simulink model "speed_control_rotativo_closed_loop"  (R2022b)
settings: Solver=VariableStepAuto  StartTime=0.0  StopTime=50  FixedStep=0.01  MaxStep=0.0005  RelTol=1e-3
libraries: simulink x5, autolibim x1, slpidlib x1
settings Model: Creator=mique  LastModifiedBy=mique

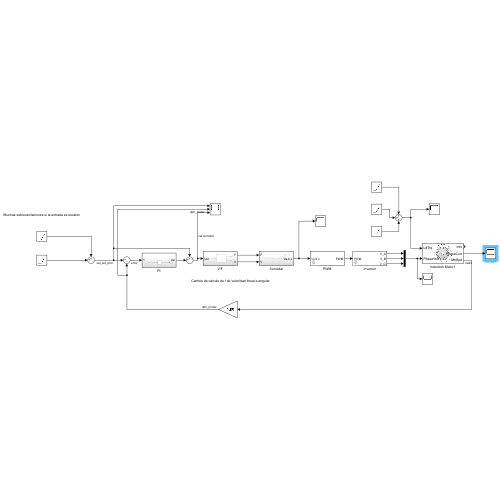
[thumbnail: Simulink's stored preview of the top-level diagram]
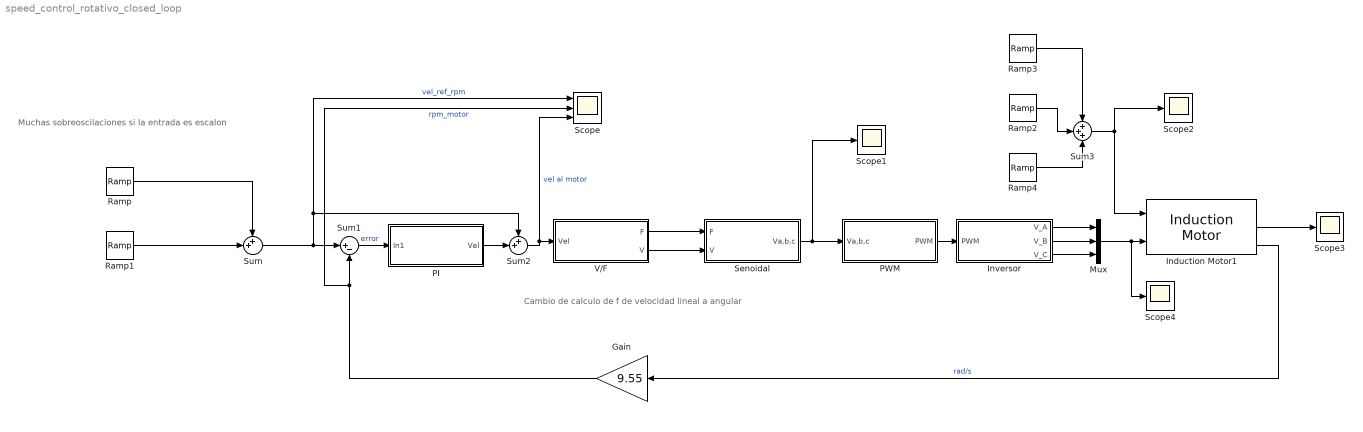
== system speed_control_rotativo_closed_loop ==
  note: Muchas sobreoscilaciones si la entrada es escalon
  note: Cambio de calculo de f de velocidad lineal a angular
  Gain : Gain  Gain=9.55
  Induction Motor1 : autolibim/Induction Motor  sim_type=Continuous  Ts=0.001  port_config=Torque  P=2  Zs=[1.77 0.0139]  Zr="[1.34  0.0121]"  Lm=0.3687  mechanical=[0.001 0 0]  theta_init=0  omega_init=0  RefBlkName='autolibim/Induction Motor'  aMode=5
      settings: LibrarySourceBlock=mcblib/Electrical Systems/Motors/Induction Motor
  Inversor : Subsystem  mask{Vmax=220}
      mask prompts: Vmax "Voltaje Maximo"
  Mux : Mux  Inputs=3
  PI : Subsystem
  PWM : Subsystem  mask{Vmax=220}
      mask prompts: Vmax "Voltaje Maximo"
  Ramp : simulink/Sources/Ramp  slope=-10  start=6  InitialOutput=0
  Ramp1 : simulink/Sources/Ramp  slope=10  start=0  InitialOutput=0
  Ramp2 : simulink/Sources/Ramp  slope=2  start=0.1  InitialOutput=0
  Ramp3 : simulink/Sources/Ramp  slope=-2  start=15  InitialOutput=0
  Ramp4 : simulink/Sources/Ramp  slope=-2  start=35  InitialOutput=0
  Scope : Scope  NumInputPorts=3
  Scope{1..4} (4 alike) : Scope
  Senoidal : Subsystem
  Sum : Sum  Inputs=++|
  Sum1 : Sum  Inputs=|+-
  Sum2 : Sum  Inputs=++|
  Sum3 : Sum  Inputs=+++
  V/F : Subsystem
  wires:
  V/F/1(F) -> Senoidal/1(F)
  Induction Motor1/2 -> Scope3/1
  Mux/1 -> Induction Motor1/2, Scope4/1
  Inversor/3(V_C) -> Mux/3
  Senoidal/1(Va,b,c) -> Scope1/1, PWM/1(Va,b,c)
  PWM/1(PWM) -> Inversor/1(PWM)
  Inversor/1(V_A) -> Mux/1
  Inversor/2(V_B) -> Mux/2
  V/F/2(V) -> Senoidal/2(V)
  Induction Motor1/3 -> Gain/1  "rad/s"
  Gain/1 -> Scope/2, Sum1/2  "rpm_motor"
  Sum/1 -> Sum2/1, Scope/1, Sum1/1  "vel_ref_rpm"
  Sum1/1 -> PI/1(In1)  "error"
  Sum2/1 -> V/F/1(Vel), Scope/3  "vel al motor"
  PI/1(Vel) -> Sum2/2
  Ramp1/1 -> Sum/2
  Ramp/1 -> Sum/1
  Ramp4/1 -> Sum3/3
  Ramp3/1 -> Sum3/1
  Sum3/1 -> Scope2/1, Induction Motor1/1
  Ramp2/1 -> Sum3/2

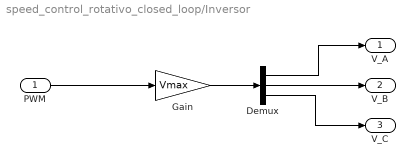
== system speed_control_rotativo_closed_loop/Inversor ==
  PWM : Inport
  Demux : Demux  Outputs=3
  Gain : Gain  Gain=Vmax
  V_A : Outport
  V_B : Outport  Port=2
  V_C : Outport  Port=3
  wires:
  PWM/1 -> Gain/1
  Demux/1 -> V_A/1
  Gain/1 -> Demux/1
  Demux/2 -> V_B/1
  Demux/3 -> V_C/1

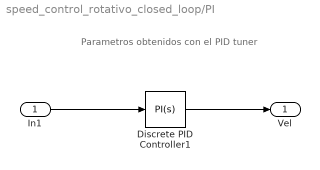
== system speed_control_rotativo_closed_loop/PI ==
  note: Parametros obtenidos con el PID tuner
  In1 : Inport
  Discrete PID Controller1 : slpidlib/PID Controller  Controller=PI  Form=Parallel  TimeDomain=Continuous-time  UseExternalTs=off  SampleTime=-1  IntegratorMethod=Forward Euler  FilterMethod=Forward Euler  ControllerParametersSource=internal  P=1  I=4.18069201960826  UseKiTs=off  D=0.0001  N=10  UseFilter=on  TunerSelectOption=Transfer Function Based (PID Tuner App)  InitialConditionSource=internal  InitialConditionForIntegrator=0  InitialConditionForFilter=0  DifferentiatorICPrevScaledInput=0  ExternalReset=none  TrackingMode=off  Kt=1  LimitOutput=off  SatLimitsSource=internal  UpperSaturationLimit=inf  LowerSaturationLimit=-inf  LinearizeAsGain=off  AntiWindupMode=none  Kb=1  LimitIntegrator=off  UpperIntegratorSaturationLimit=15  LowerIntegratorSaturationLimit=-15  POutMin=[]  POutMax=[]  IOutMin=[]  IOutMax=[]  DOutMin=[]  DOutMax=[]  NOutMin=[]  NOutMax=[]  SumOutMin=[]  SumOutMax=[]  SaturationOutMin=[]  SaturationOutMax=[]  PParamMin=[]  PParamMax=[]  IParamMin=[]  IParamMax=[]  DParamMin=[]  DParamMax=[]  NParamMin=[]  NParamMax=[]  KbParamMin=[]  KbParamMax=[]  KtParamMin=[]  KtParamMax=[]  KbOutMin=[]  KbOutMax=[]  KtOutMin=[]  KtOutMax=[]  IntegratorOutMin=[]  IntegratorOutMax=[]  FilterOutMin=[]  FilterOutMax=[]  SumI1OutMin=[]  SumI1OutMax=[]  SumI2OutMin=[]  SumI2OutMax=[]  SumI3OutMin=[]  SumI3OutMax=[]  SumI4OutMin=[]  SumI4OutMax=[]  SumDOutMin=[]  SumDOutMax=[]  DifferentiatorOutMin=[]  DifferentiatorOutMax=[]  FilterDiffOutCoefMin=[]  FilterDiffOutCoefMax=[]  ReciprocalOutMin=[]  ReciprocalOutMax=[]  SumDenOutMin=[]  SumDenOutMax=[]  SumNumOutMin=[]  SumNumOutMax=[]  DivideOutMin=[]  DivideOutMax=[]  UdiffTsProdOutMin=[]  UdiffTsProdOutMax=[]  NTsProdOutMin=[]  NTsProdOutMax=[]  UintegralTsProdOutMin=[]  UintegralTsProdOutMax=[]  UngainTsProdOutMin=[]  UngainTsProdOutMax=[]  ClampingZeroOutDataTypeStr=Inherit: Inherit via back propagation  ClampingZeroOutMin=[]  ClampingZeroOutMax=[]  FilterDenConstantOutDataTypeStr=Inherit: Inherit via back propagation  FilterDenConstantOutMin=[]  FilterDenConstantOutMax=[]  PCopyOutDataTypeStr=Inherit: Inherit via back propagation  PCopyOutMin=[]  PCopyOutMax=[]  NCopyOutDataTypeStr=Inherit: Inherit via back propagation  NCopyOutMin=[]  NCopyOutMax=[]  IntegratorContinuousStateAttributes=''  IntegratorStateMustResolveToSignalObject=off  IntegratorRTWStateStorageClass=Auto  FilterContinuousStateAttributes=''  FilterStateMustResolveToSignalObject=off  FilterRTWStateStorageClass=Auto  ParallelPVariant=InternalParameters  IdealPVariant=Disabled  IVariant=InternalParameters  DVariant=Disabled  IntegratorVariant=Continuous  SatVariant=Disabled  AWVariant=Passthrough  PCopyVariant=Disabled  TRVariant=Disabled  FdbkBlocksVariant=Forward  IdealPFdbkVariant=Disabled  SatFdbkVariant=Disabled  DerivativeFilterVariant=Disabled  NVariant=Disabled  NCopyVariant=Disabled_SignalSpec  FilterICVariant=Disabled  IntegratorICVariant=InternalICs  ExternalResetVariant=Disabled  TRSumVariant=Passthrough  SumFdbkVariant=Disabled  SumVariant=Sum_PI  TsampFilterVariant=InternalTs  TsampNgainVariant=Passthrough  TsampIntegralVariant=Passthrough  ExternalSaturationOutDataTypeStr=Inherit: Same as second input
      settings: LibrarySourceBlock=simulink/Discrete/Discrete PID Controller
  Vel : Outport
  wires:
  In1/1 -> Discrete PID Controller1/1
  Discrete PID Controller1/1 -> Vel/1

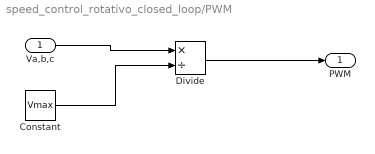
== system speed_control_rotativo_closed_loop/PWM ==
  Va,b,c : Inport
  Constant : Constant  Value=Vmax
  Divide : Product  Inputs=*/
  PWM : Outport
  wires:
  Va,b,c/1 -> Divide/1
  Constant/1 -> Divide/2
  Divide/1 -> PWM/1

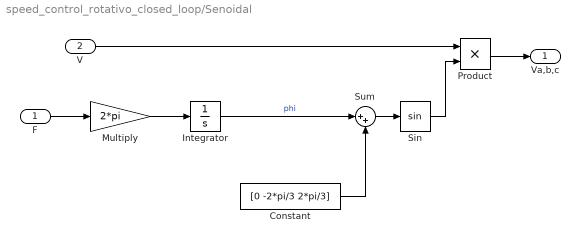
== system speed_control_rotativo_closed_loop/Senoidal ==
  F : Inport
  V : Inport  Port=2
  Constant : Constant  Value=[0 -2*pi/3 2*pi/3]
  Integrator : Integrator  WrapState=on
  Multiply : Gain  Gain=2*pi
  Product : Product
  Sin : Trigonometry
  Sum : Sum  Inputs=|++
  Va,b,c : Outport
  wires:
  Integrator/1 -> Sum/1  "phi"
  Constant/1 -> Sum/2
  Sum/1 -> Sin/1
  V/1 -> Product/1
  Sin/1 -> Product/2
  Product/1 -> Va,b,c/1
  F/1 -> Multiply/1
  Multiply/1 -> Integrator/1

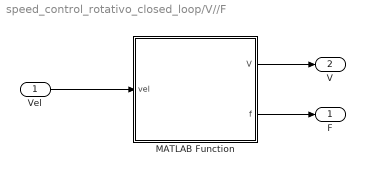
== system speed_control_rotativo_closed_loop/V//F ==
  Vel : Inport
  MATLAB Function : MATLAB Function  TreatAsAtomicUnit=on
  F : Outport
  V : Outport  Port=2
  wires:
  Vel/1 -> MATLAB Function/1(vel)
  MATLAB Function/1(V) -> V/1
  MATLAB Function/2(f) -> F/1

== matlab function speed_control_rotativo_closed_loop/V//F/MATLAB Function ==
  data: vel input; V output; f output
function [V,f]= v_f(vel)

numPolos=2;

%Velocidad en RPM
f=vel*numPolos/60;
if(f==0)
    f=0.0001;
    V=0;
    return
end

%F en HZ

%Comprobar valores
f_corte_inf=1;
V_min=40;
V_max=220;
f_corte_sup=f_corte_inf*V_max/V_min;

if(f<f_corte_inf)
    V=V_min;
    disp('zona muerta')
elseif(f<f_corte_sup)
    V=V_min/f_corte_inf*f;
    disp('zona lineal')
else
    V=V_max;
    disp('debilitamiento de campo')
end
